simulink model "examples_2"  (R2022b)
settings: Solver=VariableStepAuto  StartTime=0.0  StopTime=50  MaxStep=0.01  RelTol=1e-3
libraries: simulink x2
settings Model: Creator=Brigosha_Guest  LastModifiedBy=Brigosha_Guest

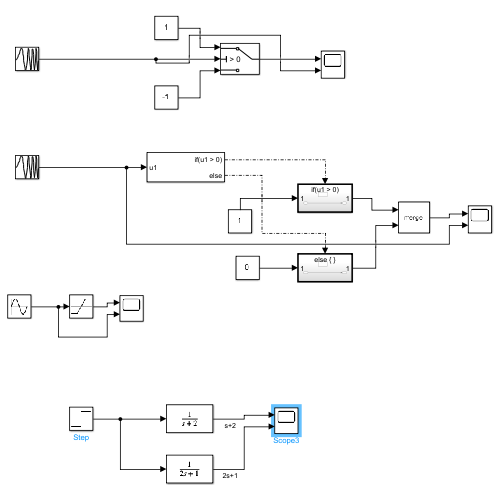
[thumbnail: Simulink's stored preview of the top-level diagram]
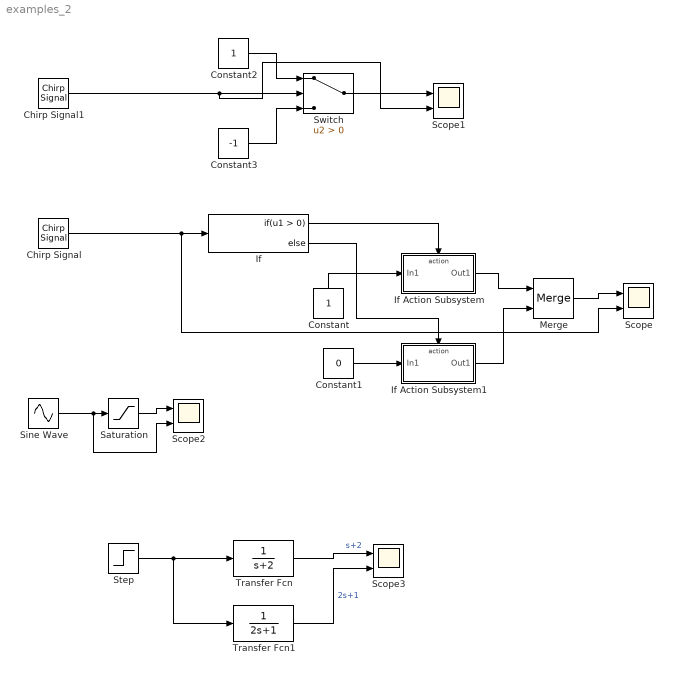
== system examples_2 ==
  Chirp Signal : simulink/Sources/Chirp Signal  f1=0.1  T=100  f2=2
  Chirp Signal1 : simulink/Sources/Chirp Signal  f1=0.1  T=100  f2=1
  Constant : Constant
  Constant1 : Constant  Value=0
  Constant2 : Constant
  Constant3 : Constant  Value=-1
  If : If
  If Action Subsystem : Subsystem  TreatAsAtomicUnit=on
  If Action Subsystem1 : Subsystem  TreatAsAtomicUnit=on
  Merge : Merge
  Saturation : Saturate
  Scope{,1..3} (4 alike) : Scope  NumInputPorts=2
  Sine Wave : Sin  SampleTime=0
  Step : Step  SampleTime=0
  Switch : Switch  Criteria=u2 > Threshold  SaturateOnIntegerOverflow=off  InputSameDT=off
  Transfer Fcn : TransferFcn  Denominator=[1 2]
  Transfer Fcn1 : TransferFcn  Denominator=[2 1]
  wires:
  Chirp Signal/1 -> Scope/2, If/1
  If/1 -> If Action Subsystem/Action
  If/2 -> If Action Subsystem1/Action
  Constant/1 -> If Action Subsystem/1(In1)
  Constant1/1 -> If Action Subsystem1/1(In1)
  If Action Subsystem/1(Out1) -> Merge/1
  If Action Subsystem1/1(Out1) -> Merge/2
  Merge/1 -> Scope/1
  Chirp Signal1/1 -> Scope1/2, Switch/2
  Constant2/1 -> Switch/1
  Constant3/1 -> Switch/3
  Switch/1 -> Scope1/1
  Sine Wave/1 -> Scope2/2, Saturation/1
  Saturation/1 -> Scope2/1
  Step/1 -> Transfer Fcn1/1, Transfer Fcn/1
  Transfer Fcn/1 -> Scope3/1  "s+2"
  Transfer Fcn1/1 -> Scope3/2  "2s+1"

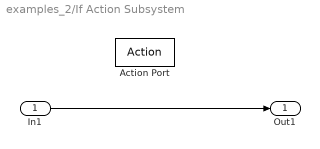
== system examples_2/If Action Subsystem ==
  In1 : Inport
  Action Port : ActionPort  ActionPortLabel=if(u1 > 0)
  Out1 : Outport
  wires:
  In1/1 -> Out1/1

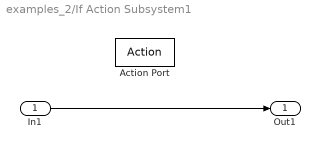
== system examples_2/If Action Subsystem1 ==
  In1 : Inport
  Action Port : ActionPort  ActionPortLabel=else
  Out1 : Outport
  wires:
  In1/1 -> Out1/1
